simulink model "simulation"  (R2022a)
settings: Solver=VariableStepAuto  StartTime=0.0  StopTime=10.0  RelTol=1e-3
values from neighbouring files (symbols this model uses):
  b = 0.00001    (= 1e-05)    [lqr_design.m]
  c = 15    [lqr_design.m]
  g = 9.81    [lqr_design.m]
  I = 5.4022e-04    (= 0.00054022)    [lqr_design.m]
  k = 4.81    [lqr_design.m]
  l = 0.147    [lqr_design.m]
  M = 0.2    [lqr_design.m]
  m = 0.075    [lqr_design.m]
  Ts = 0.02    [lqr_design.m]
undefined symbols (not defined in the file or in its folder): Kd
settings Model: Creator=raffa  LastModifiedBy=raffa

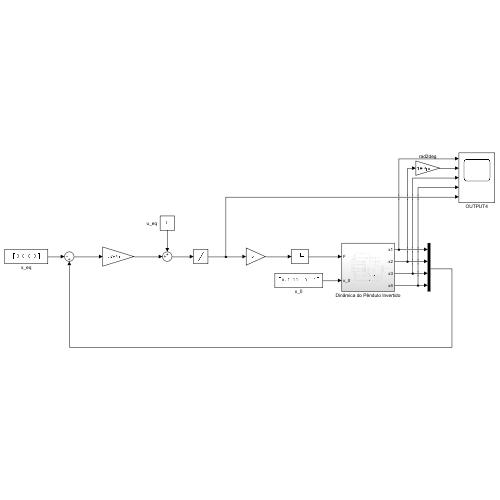
[thumbnail: Simulink's stored preview of the top-level diagram]
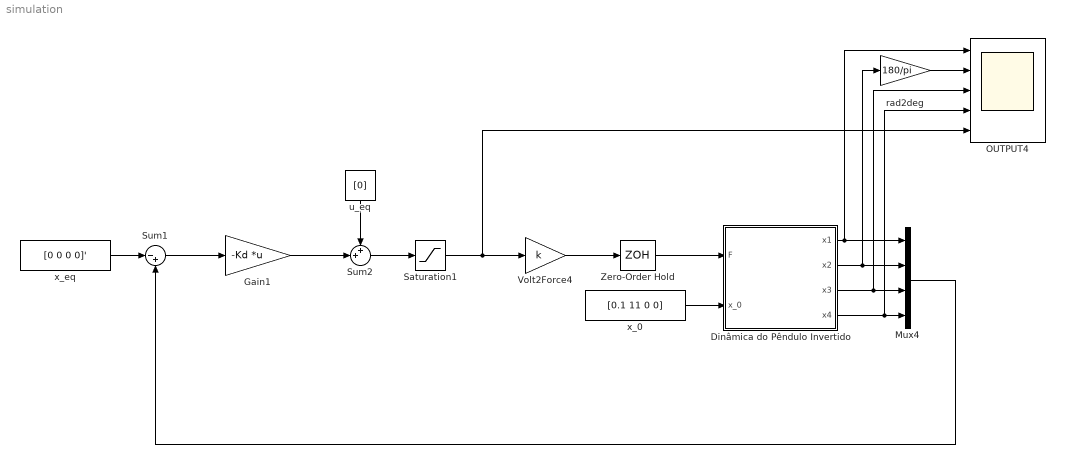
== system simulation ==
  Dinâmica do Pêndulo Invertido : Subsystem
  Gain1 : Gain  Gain=-Kd  Multiplication=Matrix(K*u)
  Mux4 : Mux
  OUTPUT4 : Scope  NumInputPorts=5
  Saturation1 : Saturate  UpperLimit=3  LowerLimit=-3
  Sum1 : Sum  Inputs=|-+
  Sum2 : Sum  Inputs=++|
  Volt2Force4 : Gain  Gain=k
  Zero-Order Hold : ZeroOrderHold  SampleTime=Ts
  rad2deg : Gain  Gain=180/pi
  u_eq : Constant  Value=[0]
  x_0 : Constant  Value=[0.1 11 0 0]
  x_eq : Constant  Value=[0 0 0 0]'
  wires:
  Sum1/1 -> Gain1/1
  rad2deg/1 -> OUTPUT4/2
  Saturation1/1 -> OUTPUT4/5, Volt2Force4/1
  u_eq/1 -> Sum2/1
  Volt2Force4/1 -> Zero-Order Hold/1
  Dinâmica do Pêndulo Invertido/4(x4) -> OUTPUT4/4, Mux4/4
  Dinâmica do Pêndulo Invertido/1(x1) -> OUTPUT4/1, Mux4/1
  Sum2/1 -> Saturation1/1
  Mux4/1 -> Sum1/2
  x_0/1 -> Dinâmica do Pêndulo Invertido/2(x_0)
  x_eq/1 -> Sum1/1
  Dinâmica do Pêndulo Invertido/3(x3) -> OUTPUT4/3, Mux4/3
  Zero-Order Hold/1 -> Dinâmica do Pêndulo Invertido/1(F)
  Dinâmica do Pêndulo Invertido/2(x2) -> rad2deg/1, Mux4/2
  Gain1/1 -> Sum2/2

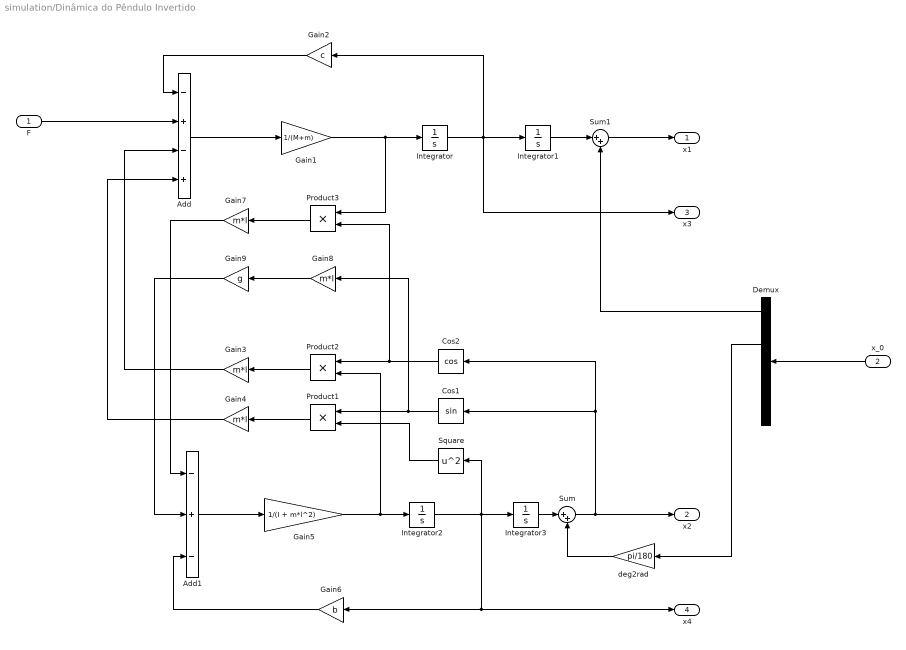
== system simulation/Dinâmica do Pêndulo Invertido ==
  F : Inport
  x_0 : Inport  Port=2
  Add : Sum  Inputs=-+-+
  Add1 : Sum  Inputs=-+-
  Cos1 : Trigonometry
  Cos2 : Trigonometry  Operator=cos
  Demux : Demux
  Gain1 : Gain  Gain=1/(M+m)
  Gain2 : Gain  Gain=c
  Gain{3..4,7..8} (4 alike) : Gain  Gain=m*l
  Gain5 : Gain  Gain=1/(I + m*l^2)
  Gain6 : Gain  Gain=b
  Gain9 : Gain  Gain=g
  Integrator{,1..3} (4 alike) : Integrator
  Product1 : Product
  Product2 : Product
  Product3 : Product
  Square : Math  Operator=square
  Sum : Sum  Inputs=|++
  Sum1 : Sum  Inputs=|++
  deg2rad : Gain  Gain=pi/180
  x1 : Outport
  x2 : Outport  Port=2
  x3 : Outport  Port=3
  x4 : Outport  Port=4
  wires:
  Cos1/1 -> Gain8/1, Product1/1
  Add/1 -> Gain1/1
  Gain5/1 -> Product2/2, Integrator2/1
  Integrator2/1 -> x4/1, Gain6/1, Square/1, Integrator3/1
  Gain3/1 -> Add/3
  Product3/1 -> Gain7/1
  Gain9/1 -> Add1/2
  Product2/1 -> Gain3/1
  Gain7/1 -> Add1/1
  Gain1/1 -> Product3/1, Integrator/1
  Gain8/1 -> Gain9/1
  Gain2/1 -> Add/1
  Integrator/1 -> x3/1, Integrator1/1, Gain2/1
  F/1 -> Add/2
  Gain4/1 -> Add/4
  Cos2/1 -> Product3/2, Product2/1
  Square/1 -> Product1/2
  Add1/1 -> Gain5/1
  Gain6/1 -> Add1/3
  Product1/1 -> Gain4/1
  Sum/1 -> x2/1, Cos2/1, Cos1/1
  Integrator3/1 -> Sum/1
  Integrator1/1 -> Sum1/1
  Sum1/1 -> x1/1
  x_0/1 -> Demux/1
  Demux/2 -> deg2rad/1
  Demux/1 -> Sum1/2
  deg2rad/1 -> Sum/2
